simulink model "schemaSIM"  (R2015b)
settings: Solver=VariableStepAuto  StartTime=0.0  StopTime=paramSIM.T  RelTol=1e-3
undefined symbols (not defined in the file or in its folder): initENG, initEST, paramENG, paramEST, paramGPS, paramIMU, paramODO
settings Model: Creator=mouyon  LastModifiedBy=mouyon

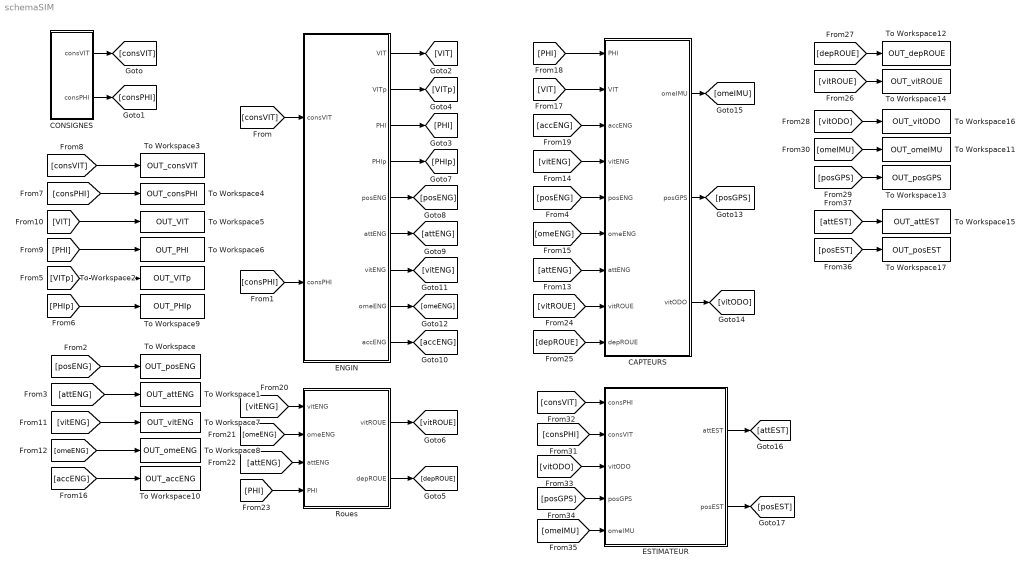
== system schemaSIM ==
  CAPTEURS : Subsystem
  CONSIGNES : Subsystem
  ENGIN : Subsystem
  ESTIMATEUR : Subsystem
  Roues : Subsystem
  To Workspace : ToWorkspace  VariableName=OUT_posENG  SaveFormat=Structure With Time  SampleTime=-1
  To Workspace1 : ToWorkspace  VariableName=OUT_attENG  SaveFormat=Structure With Time  SampleTime=-1
  To Workspace10 : ToWorkspace  VariableName=OUT_accENG  SaveFormat=Structure With Time  SampleTime=-1
  To Workspace11 : ToWorkspace  VariableName=OUT_omeIMU  SaveFormat=Structure With Time  SampleTime=-1
  To Workspace12 : ToWorkspace  VariableName=OUT_depROUE  SaveFormat=Structure With Time  SampleTime=-1
  To Workspace13 : ToWorkspace  VariableName=OUT_posGPS  SaveFormat=Structure With Time  SampleTime=-1
  To Workspace14 : ToWorkspace  VariableName=OUT_vitROUE  SaveFormat=Structure With Time  SampleTime=-1
  To Workspace15 : ToWorkspace  VariableName=OUT_attEST  SaveFormat=Structure With Time  SampleTime=-1
  To Workspace16 : ToWorkspace  VariableName=OUT_vitODO  SaveFormat=Structure With Time  SampleTime=-1
  To Workspace17 : ToWorkspace  VariableName=OUT_posEST  SaveFormat=Structure With Time  SampleTime=-1
  To Workspace2 : ToWorkspace  VariableName=OUT_VITp  SaveFormat=Structure With Time  SampleTime=-1
  To Workspace3 : ToWorkspace  VariableName=OUT_consVIT  SaveFormat=Structure With Time  SampleTime=-1
  To Workspace4 : ToWorkspace  VariableName=OUT_consPHI  SaveFormat=Structure With Time  SampleTime=-1
  To Workspace5 : ToWorkspace  VariableName=OUT_VIT  SaveFormat=Structure With Time  SampleTime=-1
  To Workspace6 : ToWorkspace  VariableName=OUT_PHI  SaveFormat=Structure With Time  SampleTime=-1
  To Workspace7 : ToWorkspace  VariableName=OUT_vitENG  SaveFormat=Structure With Time  SampleTime=-1
  To Workspace8 : ToWorkspace  VariableName=OUT_omeENG  SaveFormat=Structure With Time  SampleTime=-1
  To Workspace9 : ToWorkspace  VariableName=OUT_PHIp  SaveFormat=Structure With Time  SampleTime=-1
  wires:
  CONSIGNES/1(consVIT) -> [consVIT]
  CONSIGNES/2(consPHI) -> [consPHI]
  [consVIT] -> ENGIN/1(consVIT)
  [consPHI] -> ENGIN/2(consPHI)
  [posENG] -> To Workspace/1
  [attENG] -> To Workspace1/1
  [consVIT] -> To Workspace3/1
  [consPHI] -> To Workspace4/1
  [VIT] -> To Workspace5/1
  [PHI] -> To Workspace6/1
  [vitENG] -> To Workspace7/1
  [omeENG] -> To Workspace8/1
  ENGIN/1(VIT) -> [VIT]
  ENGIN/2(VITp) -> [VITp]
  ENGIN/3(PHI) -> [PHI]
  ENGIN/4(PHIp) -> [PHIp]
  ENGIN/6(attENG) -> [attENG]
  ENGIN/5(posENG) -> [posENG]
  ENGIN/9(accENG) -> [accENG]
  ENGIN/7(vitENG) -> [vitENG]
  [VITp] -> To Workspace2/1
  [PHIp] -> To Workspace9/1
  [accENG] -> To Workspace10/1
  [PHI] -> CAPTEURS/1(PHI)
  [VIT] -> CAPTEURS/2(VIT)
  [accENG] -> CAPTEURS/3(accENG)
  [vitENG] -> CAPTEURS/4(vitENG)
  [posENG] -> CAPTEURS/5(posENG)
  [omeENG] -> CAPTEURS/6(omeENG)
  [attENG] -> CAPTEURS/7(attENG)
  [attENG] -> Roues/3(attENG)
  [vitENG] -> Roues/1(vitENG)
  [omeENG] -> Roues/2(omeENG)
  [PHI] -> Roues/4(PHI)
  Roues/1(vitROUE) -> [vitROUE]
  Roues/2(depROUE) -> [depROUE]
  [vitROUE] -> CAPTEURS/8(vitROUE)
  [depROUE] -> CAPTEURS/9(depROUE)
  [vitROUE] -> To Workspace14/1
  [depROUE] -> To Workspace12/1
  CAPTEURS/3(vitODO) -> [vitODO]
  [vitODO] -> To Workspace16/1
  CAPTEURS/2(posGPS) -> [posGPS]
  CAPTEURS/1(omeIMU) -> [omeIMU]
  [omeIMU] -> To Workspace11/1
  ENGIN/8(omeENG) -> [omeENG]
  [posGPS] -> To Workspace13/1
  [consVIT] -> ESTIMATEUR/1(consPHI)
  [consPHI] -> ESTIMATEUR/2(consVIT)
  [vitODO] -> ESTIMATEUR/3(vitODO)
  [posGPS] -> ESTIMATEUR/4(posGPS)
  [omeIMU] -> ESTIMATEUR/5(omeIMU)
  ESTIMATEUR/1(attEST) -> [attEST]
  ESTIMATEUR/2(posEST) -> [posEST]
  [attEST] -> To Workspace15/1
  [posEST] -> To Workspace17/1

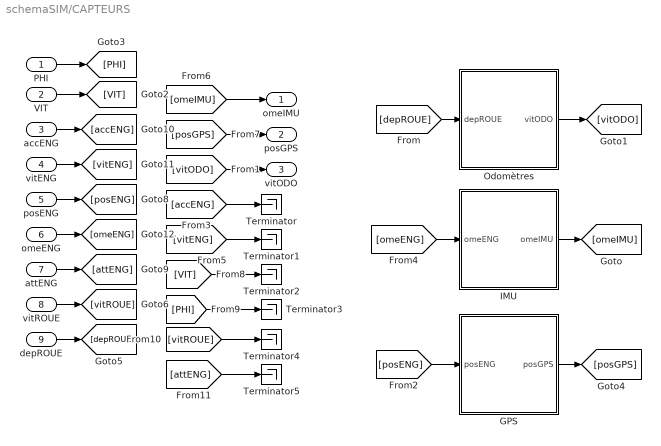
== system schemaSIM/CAPTEURS ==
  PHI : Inport
  VIT : Inport  Port=2
  accENG : Inport  Port=3
  vitENG : Inport  Port=4
  posENG : Inport  Port=5
  omeENG : Inport  Port=6
  attENG : Inport  Port=7
  vitROUE : Inport  Port=8
  depROUE : Inport  Port=9
  GPS : Subsystem
  IMU : Subsystem
  Odomètres : Subsystem
  Terminator{,1..5} (6 alike) : Terminator
  omeIMU : Outport
  posGPS : Outport  Port=2
  vitODO : Outport  Port=3
  wires:
  PHI/1 -> [PHI]
  VIT/1 -> [VIT]
  accENG/1 -> [accENG]
  vitENG/1 -> [vitENG]
  posENG/1 -> [posENG]
  omeENG/1 -> [omeENG]
  attENG/1 -> [attENG]
  vitROUE/1 -> [vitROUE]
  depROUE/1 -> [depROUE]
  [depROUE] -> Odomètres/1(depROUE)
  Odomètres/1(vitODO) -> [vitODO]
  [vitODO] -> vitODO/1
  [posGPS] -> posGPS/1
  [omeIMU] -> omeIMU/1
  [omeENG] -> IMU/1(omeENG)
  IMU/1(omeIMU) -> [omeIMU]
  [posENG] -> GPS/1(posENG)
  GPS/1(posGPS) -> [posGPS]
  [accENG] -> Terminator/1
  [vitENG] -> Terminator1/1
  [VIT] -> Terminator2/1
  [PHI] -> Terminator3/1
  [vitROUE] -> Terminator4/1
  [attENG] -> Terminator5/1

== system schemaSIM/CONSIGNES ==
  From Workspace : FromWorkspace  VariableName=IN_consVIT  SampleTime=0  Interpolate=off  OutputAfterFinalValue=Holding final value
  From Workspace1 : FromWorkspace  VariableName=IN_consPHI  SampleTime=0  Interpolate=off  OutputAfterFinalValue=Holding final value
  consVIT : Outport
  consPHI : Outport  Port=2
  wires:
  From Workspace/1 -> consVIT/1
  From Workspace1/1 -> consPHI/1

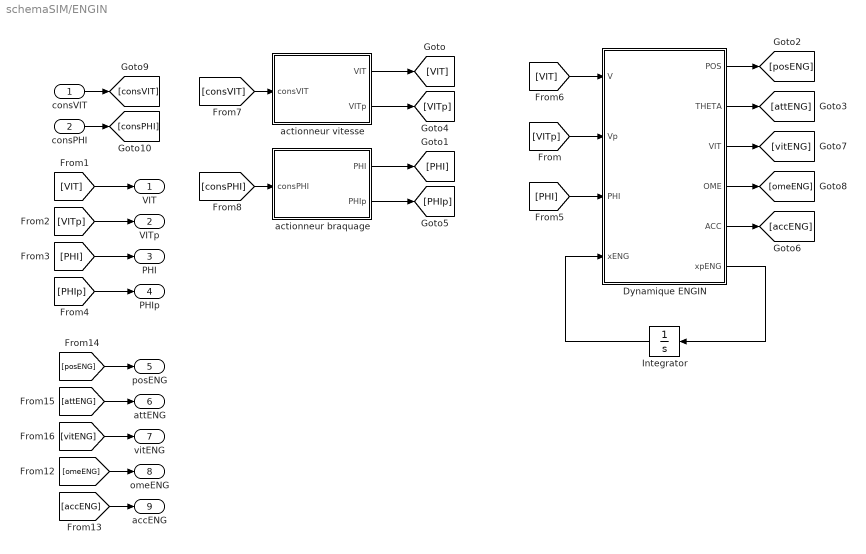
== system schemaSIM/ENGIN ==
  consVIT : Inport
  consPHI : Inport  Port=2
  Dynamique ENGIN : MATLAB Function  TreatAsAtomicUnit=on
  Integrator : Integrator  InitialCondition=initENG.x
  actionneur braquage : Subsystem
  actionneur vitesse : Subsystem
  VIT : Outport
  VITp : Outport  Port=2
  PHI : Outport  Port=3
  PHIp : Outport  Port=4
  posENG : Outport  Port=5
  attENG : Outport  Port=6
  vitENG : Outport  Port=7
  omeENG : Outport  Port=8
  accENG : Outport  Port=9
  wires:
  actionneur vitesse/1(VIT) -> [VIT]
  actionneur braquage/1(PHI) -> [PHI]
  Integrator/1 -> Dynamique ENGIN/4(xENG)
  Dynamique ENGIN/6(xpENG) -> Integrator/1
  Dynamique ENGIN/1(POS) -> [posENG]
  Dynamique ENGIN/2(THETA) -> [attENG]
  [VIT] -> Dynamique ENGIN/1(V)
  [PHI] -> Dynamique ENGIN/3(PHI)
  Dynamique ENGIN/3(VIT) -> [vitENG]
  Dynamique ENGIN/4(OME) -> [omeENG]
  actionneur vitesse/2(VITp) -> [VITp]
  actionneur braquage/2(PHIp) -> [PHIp]
  [VITp] -> Dynamique ENGIN/2(Vp)
  Dynamique ENGIN/5(ACC) -> [accENG]
  [VIT] -> VIT/1
  [VITp] -> VITp/1
  [PHI] -> PHI/1
  [PHIp] -> PHIp/1
  [posENG] -> posENG/1
  [attENG] -> attENG/1
  [vitENG] -> vitENG/1
  [omeENG] -> omeENG/1
  [accENG] -> accENG/1
  consVIT/1 -> [consVIT]
  consPHI/1 -> [consPHI]
  [consVIT] -> actionneur vitesse/1(consVIT)
  [consPHI] -> actionneur braquage/1(consPHI)

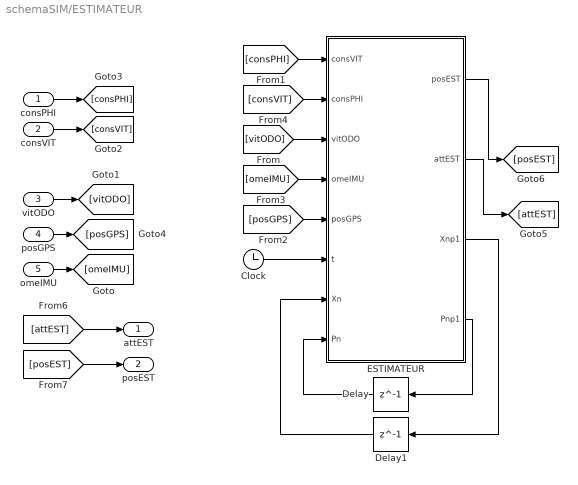
== system schemaSIM/ESTIMATEUR ==
  consPHI : Inport
  consVIT : Inport  Port=2
  vitODO : Inport  Port=3
  posGPS : Inport  Port=4
  omeIMU : Inport  Port=5
  Clock : Clock
  Delay : Delay  DelayLength=1  InitialCondition=initEST.P  SampleTime=paramEST.dt
  Delay1 : Delay  DelayLength=1  InitialCondition=initEST.x  SampleTime=paramEST.dt
  ESTIMATEUR : MATLAB Function  TreatAsAtomicUnit=on
  attEST : Outport
  posEST : Outport  Port=2
  wires:
  consPHI/1 -> [consPHI]
  consVIT/1 -> [consVIT]
  vitODO/1 -> [vitODO]
  posGPS/1 -> [posGPS]
  omeIMU/1 -> [omeIMU]
  [posEST] -> posEST/1
  [attEST] -> attEST/1
  [vitODO] -> ESTIMATEUR/3(vitODO)
  [omeIMU] -> ESTIMATEUR/4(omeIMU)
  [posGPS] -> ESTIMATEUR/5(posGPS)
  Clock/1 -> ESTIMATEUR/6(t)
  ESTIMATEUR/4(Pnp1) -> Delay/1
  ESTIMATEUR/3(Xnp1) -> Delay1/1
  ESTIMATEUR/1(posEST) -> [posEST]
  ESTIMATEUR/2(attEST) -> [attEST]
  Delay1/1 -> ESTIMATEUR/7(Xn)
  Delay/1 -> ESTIMATEUR/8(Pn)
  [consPHI] -> ESTIMATEUR/1(consVIT)
  [consVIT] -> ESTIMATEUR/2(consPHI)

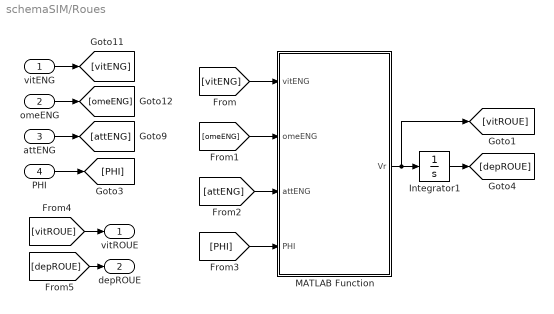
== system schemaSIM/Roues ==
  vitENG : Inport
  omeENG : Inport  Port=2
  attENG : Inport  Port=3
  PHI : Inport  Port=4
  Integrator1 : Integrator  InitialCondition=zeros(4,1)
  MATLAB Function : MATLAB Function  TreatAsAtomicUnit=on
  vitROUE : Outport
  depROUE : Outport  Port=2
  wires:
  [vitENG] -> MATLAB Function/1(vitENG)
  [omeENG] -> MATLAB Function/2(omeENG)
  [attENG] -> MATLAB Function/3(attENG)
  [PHI] -> MATLAB Function/4(PHI)
  MATLAB Function/1(Vr) -> [vitROUE], Integrator1/1
  Integrator1/1 -> [depROUE]
  vitENG/1 -> [vitENG]
  omeENG/1 -> [omeENG]
  attENG/1 -> [attENG]
  PHI/1 -> [PHI]
  [vitROUE] -> vitROUE/1
  [depROUE] -> depROUE/1

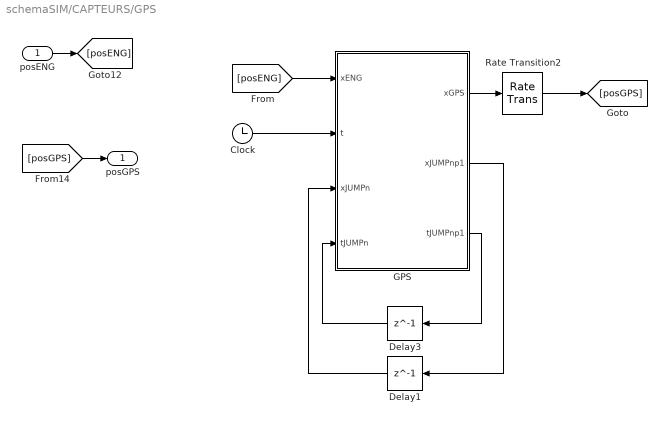
== system schemaSIM/CAPTEURS/GPS ==
  posENG : Inport
  Clock : Clock
  Delay1 : Delay  DelayLength=1  InitialCondition=zeros(2,1)  SampleTime=paramGPS.dt
  Delay3 : Delay  DelayLength=1  InitialCondition=paramGPS.per_sau*rand  SampleTime=paramGPS.dt
  GPS : MATLAB Function  TreatAsAtomicUnit=on
  Rate Transition2 : RateTransition  OutPortSampleTime=paramGPS.dt
  posGPS : Outport
  wires:
  [posGPS] -> posGPS/1
  posENG/1 -> [posENG]
  Clock/1 -> GPS/2(t)
  GPS/1(xGPS) -> Rate Transition2/1
  GPS/3(tJUMPnp1) -> Delay3/1
  Delay3/1 -> GPS/4(tJUMPn)
  GPS/2(xJUMPnp1) -> Delay1/1
  Delay1/1 -> GPS/3(xJUMPn)
  Rate Transition2/1 -> [posGPS]
  [posENG] -> GPS/1(xENG)

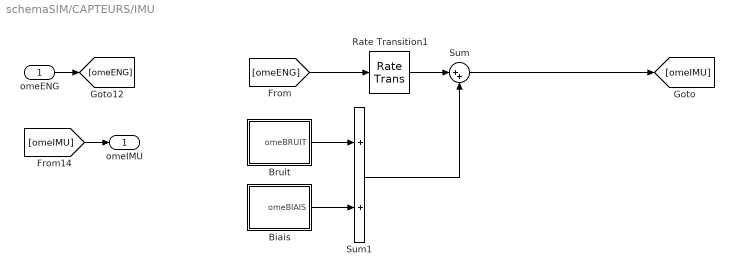
== system schemaSIM/CAPTEURS/IMU ==
  omeENG : Inport
  Biais : Subsystem
  Bruit : Subsystem
  Rate Transition1 : RateTransition  OutPortSampleTime=paramIMU.dt
  Sum : Sum  Inputs=|++
  Sum1 : Sum
  omeIMU : Outport
  wires:
  [omeIMU] -> omeIMU/1
  omeENG/1 -> [omeENG]
  [omeENG] -> Rate Transition1/1
  Rate Transition1/1 -> Sum/1
  Bruit/1(omeBRUIT) -> Sum1/1
  Biais/1(omeBIAIS) -> Sum1/2
  Sum1/1 -> Sum/2
  Sum/1 -> [omeIMU]

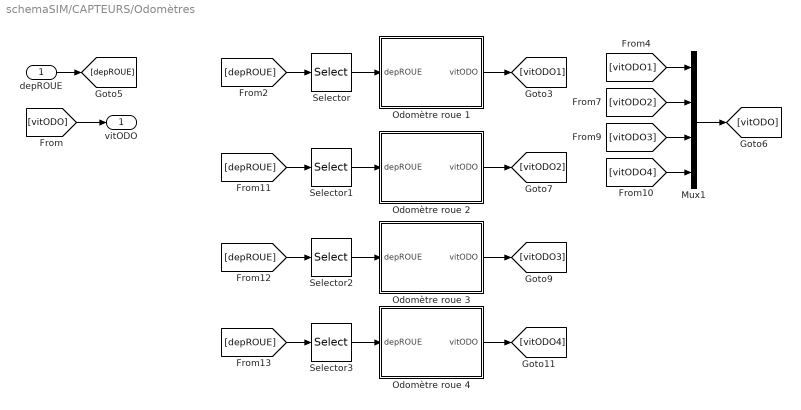
== system schemaSIM/CAPTEURS/Odomètres ==
  depROUE : Inport
  Mux1 : Mux
  Odomètre roue 1 : Subsystem
  Odomètre roue 2 : Subsystem
  Odomètre roue 3 : Subsystem
  Odomètre roue 4 : Subsystem
  Selector : Selector  InputPortWidth=4  IndexOptions=Index vector (dialog)  Indices=[1]  OutputSizes=1
  Selector1 : Selector  InputPortWidth=4  IndexOptions=Index vector (dialog)  Indices=[2]  OutputSizes=1
  Selector2 : Selector  InputPortWidth=4  IndexOptions=Index vector (dialog)  Indices=[3]  OutputSizes=1
  Selector3 : Selector  InputPortWidth=4  IndexOptions=Index vector (dialog)  Indices=[4]  OutputSizes=1
  vitODO : Outport
  wires:
  depROUE/1 -> [depROUE]
  [vitODO] -> vitODO/1
  [depROUE] -> Selector/1
  Selector/1 -> Odomètre roue 1/1(depROUE)
  Odomètre roue 1/1(vitODO) -> [vitODO1]
  Mux1/1 -> [vitODO]
  [vitODO1] -> Mux1/1
  [vitODO2] -> Mux1/2
  [vitODO3] -> Mux1/3
  [vitODO4] -> Mux1/4
  [depROUE] -> Selector1/1
  Selector1/1 -> Odomètre roue 2/1(depROUE)
  Odomètre roue 2/1(vitODO) -> [vitODO2]
  [depROUE] -> Selector2/1
  Selector2/1 -> Odomètre roue 3/1(depROUE)
  Odomètre roue 3/1(vitODO) -> [vitODO3]
  [depROUE] -> Selector3/1
  Selector3/1 -> Odomètre roue 4/1(depROUE)
  Odomètre roue 4/1(vitODO) -> [vitODO4]

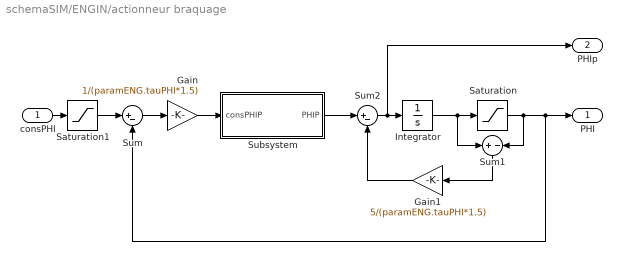
== system schemaSIM/ENGIN/actionneur braquage ==
  consPHI : Inport
  Gain : Gain  Gain=1/(paramENG.tauPHI*1.5)
  Gain1 : Gain  Gain=5/(paramENG.tauPHI*1.5)
  Integrator : Integrator  InitialCondition=initENG.PHI
  Saturation : Saturate  UpperLimit=paramENG.maxPHI  LowerLimit=-paramENG.maxPHI
  Saturation1 : Saturate  UpperLimit=paramENG.maxPHI  LowerLimit=-paramENG.maxPHI
  Subsystem : Subsystem
  Sum : Sum  Inputs=|+-
  Sum1 : Sum  Inputs=+|-
  Sum2 : Sum  Inputs=|+-
  PHI : Outport
  PHIp : Outport  Port=2
  wires:
  Integrator/1 -> Sum1/1, Saturation/1
  consPHI/1 -> Saturation1/1
  Sum/1 -> Gain/1
  Saturation/1 -> Sum1/2, PHI/1, Sum/2
  Sum1/1 -> Gain1/1
  Gain1/1 -> Sum2/2
  Sum2/1 -> PHIp/1, Integrator/1
  Gain/1 -> Subsystem/1(consPHIP)
  Subsystem/1(PHIP) -> Sum2/1
  Saturation1/1 -> Sum/1

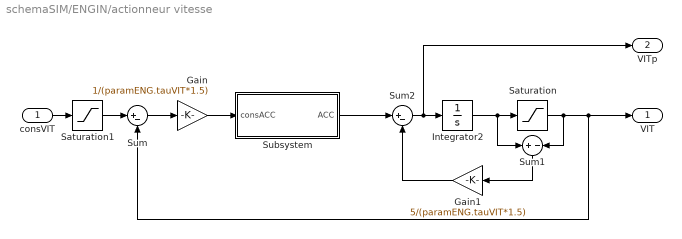
== system schemaSIM/ENGIN/actionneur vitesse ==
  consVIT : Inport
  Gain : Gain  Gain=1/(paramENG.tauVIT*1.5)
  Gain1 : Gain  Gain=5/(paramENG.tauVIT*1.5)
  Integrator2 : Integrator  InitialCondition=initENG.VIT
  Saturation : Saturate  UpperLimit=paramENG.maxVIT  LowerLimit=paramENG.minVIT
  Saturation1 : Saturate  UpperLimit=paramENG.maxVIT  LowerLimit=paramENG.minVIT
  Subsystem : Subsystem
  Sum : Sum  Inputs=|+-
  Sum1 : Sum  Inputs=+|-
  Sum2 : Sum  Inputs=|+-
  VIT : Outport
  VITp : Outport  Port=2
  wires:
  Integrator2/1 -> Sum1/1, Saturation/1
  consVIT/1 -> Saturation1/1
  Sum/1 -> Gain/1
  Saturation/1 -> Sum1/2, VIT/1, Sum/2
  Sum1/1 -> Gain1/1
  Gain1/1 -> Sum2/2
  Sum2/1 -> VITp/1, Integrator2/1
  Gain/1 -> Subsystem/1(consACC)
  Subsystem/1(ACC) -> Sum2/1
  Saturation1/1 -> Sum/1

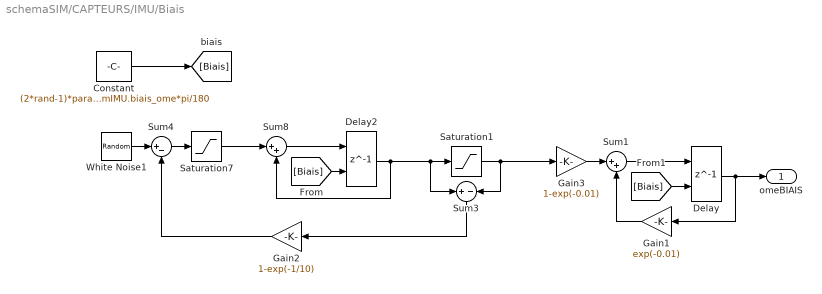
== system schemaSIM/CAPTEURS/IMU/Biais ==
  Constant : Constant  Value=(2*rand-1)*paramIMU.biais_ome*pi/180
  Delay : Delay  DelayLength=1  InitialConditionSource=Input port  InitialCondition=0
      settings: InputPortMap=u0,p4
  Delay2 : Delay  DelayLength=1  InitialConditionSource=Input port  InitialCondition=0
      settings: InputPortMap=u0,p4
  Gain1 : Gain  Gain=exp(-0.01)
  Gain2 : Gain  Gain=1-exp(-1/10)
  Gain3 : Gain  Gain=1-exp(-0.01)
  Saturation1 : Saturate  UpperLimit=paramIMU.biais_ome*pi/180  LowerLimit=-paramIMU.biais_ome*pi/180
  Saturation7 : Saturate  UpperLimit=paramIMU.deriv_ome*pi/180*paramIMU.dt  LowerLimit=-paramIMU.deriv_ome*pi/180*paramIMU.dt
  Sum1 : Sum  Inputs=|++
  Sum3 : Sum  Inputs=+|-
  Sum4 : Sum  Inputs=|+-
  Sum8 : Sum  Inputs=|++
  White Noise1 : RandomNumber  DisableCoverage=on  Variance=0.995*(paramIMU.biais_ome*pi/180/3)^2  SampleTime=paramIMU.dt
  omeBIAIS : Outport
  wires:
  Constant/1 -> [Biais]
  Delay/1 -> omeBIAIS/1, Gain1/1
  Sum1/1 -> Delay/1
  [Biais] -> Delay/2
  Gain3/1 -> Sum1/1
  Gain1/1 -> Sum1/2
  Sum3/1 -> Gain2/1
  Gain2/1 -> Sum4/2
  White Noise1/1 -> Sum4/1
  [Biais] -> Delay2/2
  Sum8/1 -> Delay2/1
  Sum4/1 -> Saturation7/1
  Delay2/1 -> Sum3/1, Saturation1/1, Sum8/2
  Saturation1/1 -> Gain3/1, Sum3/2
  Saturation7/1 -> Sum8/1

== system schemaSIM/CAPTEURS/IMU/Bruit ==
  White Noise : RandomNumber  DisableCoverage=on  Variance=(paramIMU.sig_ome*pi/180)^2  SampleTime=paramIMU.dt
  omeBRUIT : Outport
  wires:
  White Noise/1 -> omeBRUIT/1

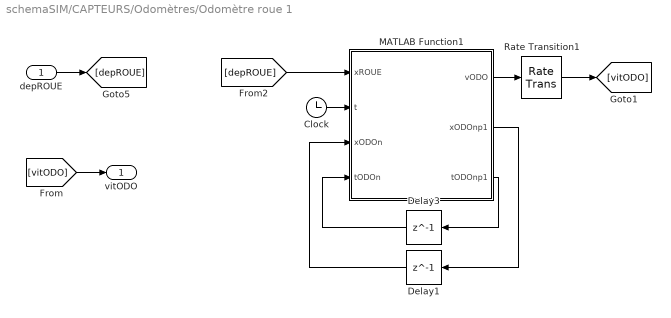
== system schemaSIM/CAPTEURS/Odomètres/Odomètre roue 1 ==
  depROUE : Inport
  Clock : Clock
  Delay1 : Delay  DelayLength=1  InitialCondition=0  SampleTime=paramODO.dt
  Delay3 : Delay  DelayLength=1  InitialCondition=0  SampleTime=paramODO.dt
  MATLAB Function1 : MATLAB Function  TreatAsAtomicUnit=on
  Rate Transition1 : RateTransition  OutPortSampleTime=paramODO.dt
  vitODO : Outport
  wires:
  Clock/1 -> MATLAB Function1/2(t)
  MATLAB Function1/1(vODO) -> Rate Transition1/1
  Rate Transition1/1 -> [vitODO]
  MATLAB Function1/3(tODOnp1) -> Delay3/1
  Delay3/1 -> MATLAB Function1/4(tODOn)
  MATLAB Function1/2(xODOnp1) -> Delay1/1
  Delay1/1 -> MATLAB Function1/3(xODOn)
  depROUE/1 -> [depROUE]
  [depROUE] -> MATLAB Function1/1(xROUE)
  [vitODO] -> vitODO/1

== system schemaSIM/CAPTEURS/Odomètres/Odomètre roue 2 ==
  depROUE : Inport
  Clock : Clock
  Delay1 : Delay  DelayLength=1  InitialCondition=0  SampleTime=paramODO.dt
  Delay3 : Delay  DelayLength=1  InitialCondition=0  SampleTime=paramODO.dt
  MATLAB Function1 : MATLAB Function  TreatAsAtomicUnit=on
  Rate Transition1 : RateTransition  OutPortSampleTime=paramODO.dt
  vitODO : Outport
  wires:
  Clock/1 -> MATLAB Function1/2(t)
  MATLAB Function1/1(vODO) -> Rate Transition1/1
  Rate Transition1/1 -> [vitODO]
  MATLAB Function1/3(tODOnp1) -> Delay3/1
  Delay3/1 -> MATLAB Function1/4(tODOn)
  MATLAB Function1/2(xODOnp1) -> Delay1/1
  Delay1/1 -> MATLAB Function1/3(xODOn)
  depROUE/1 -> [depROUE]
  [depROUE] -> MATLAB Function1/1(xROUE)
  [vitODO] -> vitODO/1

== system schemaSIM/CAPTEURS/Odomètres/Odomètre roue 3 ==
  depROUE : Inport
  Clock : Clock
  Delay1 : Delay  DelayLength=1  InitialCondition=0  SampleTime=paramODO.dt
  Delay3 : Delay  DelayLength=1  InitialCondition=0  SampleTime=paramODO.dt
  MATLAB Function1 : MATLAB Function  TreatAsAtomicUnit=on
  Rate Transition1 : RateTransition  OutPortSampleTime=paramODO.dt
  vitODO : Outport
  wires:
  Clock/1 -> MATLAB Function1/2(t)
  MATLAB Function1/1(vODO) -> Rate Transition1/1
  Rate Transition1/1 -> [vitODO]
  MATLAB Function1/3(tODOnp1) -> Delay3/1
  Delay3/1 -> MATLAB Function1/4(tODOn)
  MATLAB Function1/2(xODOnp1) -> Delay1/1
  Delay1/1 -> MATLAB Function1/3(xODOn)
  depROUE/1 -> [depROUE]
  [depROUE] -> MATLAB Function1/1(xROUE)
  [vitODO] -> vitODO/1

== system schemaSIM/CAPTEURS/Odomètres/Odomètre roue 4 ==
  depROUE : Inport
  Clock : Clock
  Delay1 : Delay  DelayLength=1  InitialCondition=0  SampleTime=paramODO.dt
  Delay3 : Delay  DelayLength=1  InitialCondition=0  SampleTime=paramODO.dt
  MATLAB Function1 : MATLAB Function  TreatAsAtomicUnit=on
  Rate Transition1 : RateTransition  OutPortSampleTime=paramODO.dt
  vitODO : Outport
  wires:
  Clock/1 -> MATLAB Function1/2(t)
  MATLAB Function1/1(vODO) -> Rate Transition1/1
  Rate Transition1/1 -> [vitODO]
  MATLAB Function1/3(tODOnp1) -> Delay3/1
  Delay3/1 -> MATLAB Function1/4(tODOn)
  MATLAB Function1/2(xODOnp1) -> Delay1/1
  Delay1/1 -> MATLAB Function1/3(xODOn)
  depROUE/1 -> [depROUE]
  [depROUE] -> MATLAB Function1/1(xROUE)
  [vitODO] -> vitODO/1

== system schemaSIM/ENGIN/actionneur braquage/Subsystem ==
  consPHIP : Inport
  Gain2 : Gain  Gain=5/(paramENG.tauPHI/1.5)
  Gain3 : Gain  Gain=1/(paramENG.tauPHI/1.5)
  Integrator1 : Integrator
  Saturation1 : Saturate  UpperLimit=paramENG.maxPHIP  LowerLimit=-paramENG.maxPHIP
  Saturation2 : Saturate  UpperLimit=paramENG.maxPHIP  LowerLimit=-paramENG.maxPHIP
  Sum3 : Sum  Inputs=+|-
  Sum4 : Sum  Inputs=|+-
  Sum5 : Sum  Inputs=|+-
  PHIP : Outport
  wires:
  Integrator1/1 -> Sum3/1, Saturation1/1
  Sum3/1 -> Gain2/1
  Gain2/1 -> Sum4/2
  Sum4/1 -> Integrator1/1
  Gain3/1 -> Sum4/1
  Saturation1/1 -> PHIP/1, Sum5/2, Sum3/2
  Sum5/1 -> Gain3/1
  consPHIP/1 -> Saturation2/1
  Saturation2/1 -> Sum5/1

== system schemaSIM/ENGIN/actionneur vitesse/Subsystem ==
  consACC : Inport
  Gain2 : Gain  Gain=5/(paramENG.tauVIT/1.5)
  Gain3 : Gain  Gain=1/(paramENG.tauVIT/1.5)
  Integrator1 : Integrator
  Saturation1 : Saturate  UpperLimit=paramENG.maxVITP  LowerLimit=-paramENG.maxVITP
  Saturation2 : Saturate  UpperLimit=paramENG.maxVITP  LowerLimit=-paramENG.maxVITP
  Sum3 : Sum  Inputs=+|-
  Sum4 : Sum  Inputs=|+-
  Sum5 : Sum  Inputs=|+-
  ACC : Outport
  wires:
  Integrator1/1 -> Sum3/1, Saturation1/1
  Sum3/1 -> Gain2/1
  Gain2/1 -> Sum4/2
  Sum4/1 -> Integrator1/1
  Gain3/1 -> Sum4/1
  Saturation1/1 -> ACC/1, Sum5/2, Sum3/2
  Sum5/1 -> Gain3/1
  consACC/1 -> Saturation2/1
  Saturation2/1 -> Sum5/1

== matlab function schemaSIM/CAPTEURS/Odomètres/Odomètre roue 2/MATLAB Function1 ==
  data: xROUE input size=1; t input size=1; xODOn input size=1; tODOn input size=1; vODO output size=1; xODOnp1 output size=1; paramODO parameter; tODOnp1 output size=1
function [vODO,xODOnp1,tODOnp1]  = Odometre(xROUE,t,xODOn,tODOn,paramODO)

% [vODO,xODOnp1,tODOnp1]  = Odometre(xROUE,t,xODOn,tODOn,paramODO);
%--------------------------------------------------------------------------
%   xROUE :	position courante de la roue 
%   t :     date courante
%   xODOn :	position au top précédent
%   tODOn :	date au top précédent
% 
%   vitODO :    vitesse mesurée 
%   xODOnp1 :	position au dernier top 
%   tODOnp1 :	date au dernier top
%--------------------------------------------------------------------------

% Paramètres
dx	= paramODO.dx;
sig	= paramODO.sig_vit;

% Variations
Dx = xROUE-xODOn;
Dt = t-tODOn;

% Incrément du nombre de TOP
nTOP = fix(Dx/dx);

% Déplacement quantifié (pas dx)
dxODO = nTOP*dx;

% Ajout incertitude de mesure
dxINC = sig*Dt*randn;
dxODO = dxODO + dxINC;

% Déplacement mesuré
if nTOP~=0
    % Au moins un TOP reçu
    xODOnp1 = xODOn + dxODO;
    tODOnp1  = t;
else
    % Aucun TOP reçu
    xODOnp1 = xODOn;
    tODOnp1 = tODOn;
end;

% Vitesse mesurée
vODO = (xODOnp1-xODOn)*Dt/(Dt*Dt+eps);

== matlab function schemaSIM/CAPTEURS/Odomètres/Odomètre roue 1/MATLAB Function1 ==
  data: xROUE input size=1; t input size=1; xODOn input size=1; tODOn input size=1; vODO output size=1; xODOnp1 output size=1; paramODO parameter; tODOnp1 output size=1
function [vODO,xODOnp1,tODOnp1]  = Odometre(xROUE,t,xODOn,tODOn,paramODO)

% [vODO,xODOnp1,tODOnp1]  = Odometre(xROUE,t,xODOn,tODOn,paramODO);
%--------------------------------------------------------------------------
%   xROUE :	position courante de la roue 
%   t :     date courante
%   xODOn :	position au top précédent
%   tODOn :	date au top précédent
% 
%   vitODO :    vitesse mesurée 
%   xODOnp1 :	position au dernier top 
%   tODOnp1 :	date au dernier top
%--------------------------------------------------------------------------

% Paramètres
dx	= paramODO.dx;
sig	= paramODO.sig_vit;

% Variations
Dx = xROUE-xODOn;
Dt = t-tODOn;

% Incrément du nombre de TOP
nTOP = fix(Dx/dx);

% Déplacement quantifié (pas dx)
dxODO = nTOP*dx;

% Ajout incertitude de mesure
dxINC = sig*Dt*randn;
dxODO = dxODO + dxINC;

% Déplacement mesuré
if nTOP~=0
    % Au moins un TOP reçu
    xODOnp1 = xODOn + dxODO;
    tODOnp1  = t;
else
    % Aucun TOP reçu
    xODOnp1 = xODOn;
    tODOnp1 = tODOn;
end;

% Vitesse mesurée
vODO = (xODOnp1-xODOn)*Dt/(Dt*Dt+eps);

== matlab function schemaSIM/ENGIN/Dynamique ENGIN ==
  data: V input size=1; Vp input; POS output size=2; THETA output size=1; VIT output; OME output; ACC output; PHI input size=1; xENG input size=initENG.nx; xpENG output size=initENG.nx; paramENG parameter
function [POS,THETA,VIT,OME,ACC,xpENG] = dynENGIN(V,Vp,PHI,xENG,paramENG)

% [POS,THETA,VIT,OME,ACC,xpENG] = dynENGIN(V,Vp,PHI,xENG,paramENG);
%--------------------------------------------------------------------------
% POS: position centre essieu arrière
% THETA: cap
% VIT: vitesse du centre de l'essieu arrière
% OME: vitesse de rotation
% ACC: accélération du centre de l'essieu arrière
%--------------------------------------------------------------------------
% WARNING: PHI est en degrés 
%--------------------------------------------------------------------------

% Decodage des arguments d'entree
x       = xENG(1);  % [m]
y       = xENG(2);  % [m]
the     = xENG(3);  % [rd]
phi     = PHI*pi/180;

% Dynamique de l'état
xp      = V * cos(the);
yp      = V * sin(the);
attp	= V/paramENG.L * tan(phi);

% Accélération
Vxp     = Vp * cos(the) - V^2 * tan(phi) * sin(the);
Vyp     = Vp * sin(the) + V^2 * tan(phi) * cos(the);

% Encodage des arguments de sortie
POS     = [x;y];
THETA	= [the];
VIT     = [xp;yp];
OME     = [attp];
ACC     = [Vxp;Vyp];
xpENG	= [xp;yp;attp];

== matlab function schemaSIM/CAPTEURS/Odomètres/Odomètre roue 3/MATLAB Function1 ==
  data: xROUE input size=1; t input size=1; xODOn input size=1; tODOn input size=1; vODO output size=1; xODOnp1 output size=1; paramODO parameter; tODOnp1 output size=1
function [vODO,xODOnp1,tODOnp1]  = Odometre(xROUE,t,xODOn,tODOn,paramODO)

% [vODO,xODOnp1,tODOnp1]  = Odometre(xROUE,t,xODOn,tODOn,paramODO);
%--------------------------------------------------------------------------
%   xROUE :	position courante de la roue 
%   t :     date courante
%   xODOn :	position au top précédent
%   tODOn :	date au top précédent
% 
%   vitODO :    vitesse mesurée 
%   xODOnp1 :	position au dernier top 
%   tODOnp1 :	date au dernier top
%--------------------------------------------------------------------------

% Paramètres
dx	= paramODO.dx;
sig	= paramODO.sig_vit;

% Variations
Dx = xROUE-xODOn;
Dt = t-tODOn;

% Incrément du nombre de TOP
nTOP = fix(Dx/dx);

% Déplacement quantifié (pas dx)
dxODO = nTOP*dx;

% Ajout incertitude de mesure
dxINC = sig*Dt*randn;
dxODO = dxODO + dxINC;

% Déplacement mesuré
if nTOP~=0
    % Au moins un TOP reçu
    xODOnp1 = xODOn + dxODO;
    tODOnp1  = t;
else
    % Aucun TOP reçu
    xODOnp1 = xODOn;
    tODOnp1 = tODOn;
end;

% Vitesse mesurée
vODO = (xODOnp1-xODOn)*Dt/(Dt*Dt+eps);

== matlab function schemaSIM/CAPTEURS/Odomètres/Odomètre roue 4/MATLAB Function1 ==
  data: xROUE input size=1; t input size=1; xODOn input size=1; tODOn input size=1; vODO output size=1; xODOnp1 output size=1; paramODO parameter; tODOnp1 output size=1
function [vODO,xODOnp1,tODOnp1]  = Odometre(xROUE,t,xODOn,tODOn,paramODO)

% [vODO,xODOnp1,tODOnp1]  = Odometre(xROUE,t,xODOn,tODOn,paramODO);
%--------------------------------------------------------------------------
%   xROUE :	position courante de la roue 
%   t :     date courante
%   xODOn :	position au top précédent
%   tODOn :	date au top précédent
% 
%   vitODO :    vitesse mesurée 
%   xODOnp1 :	position au dernier top 
%   tODOnp1 :	date au dernier top
%--------------------------------------------------------------------------

% Paramètres
dx	= paramODO.dx;
sig	= paramODO.sig_vit;

% Variations
Dx = xROUE-xODOn;
Dt = t-tODOn;

% Incrément du nombre de TOP
nTOP = fix(Dx/dx);

% Déplacement quantifié (pas dx)
dxODO = nTOP*dx;

% Ajout incertitude de mesure
dxINC = sig*Dt*randn;
dxODO = dxODO + dxINC;

% Déplacement mesuré
if nTOP~=0
    % Au moins un TOP reçu
    xODOnp1 = xODOn + dxODO;
    tODOnp1  = t;
else
    % Aucun TOP reçu
    xODOnp1 = xODOn;
    tODOnp1 = tODOn;
end;

% Vitesse mesurée
vODO = (xODOnp1-xODOn)*Dt/(Dt*Dt+eps);

== matlab function schemaSIM/Roues/MATLAB Function ==
  data: vitENG input size=2; omeENG input size=1; Vr output size=4; attENG input size=1; PHI input size=1; paramENG parameter
function Vr  = vitROUE(vitENG,omeENG,attENG,PHI,paramENG)

% Vr = vitROUE(vitENG,omeENG,attENG,PHI,paramENG);
%--------------------------------------------------------------------------
% Vr(1): vitesse roue arrière gauche
% Vr(2): vitesse roue arrière droite
% Vr(3): vitesse roue avant gauche
% Vr(4): vitesse roue avant droite
%--------------------------------------------------------------------------
% WARNING: PHI est en degrés 
%--------------------------------------------------------------------------

% Decodage des arguments d'entree
Vx      = vitENG(1);
Vy      = vitENG(2);
omega	= omeENG;
theta	= attENG;
phi     = PHI*pi/180;

% Paramètres
H   = paramENG.H;
L	= paramENG.L;

% Vitesses (de roulement) des roues
Vr = zeros(4,1);
Vr(1,1) = cos(theta)*Vx + sin(theta)*Vy - omega*H;
Vr(2,1) = cos(theta)*Vx + sin(theta)*Vy + omega*H;
Vr(3,1) = cos(theta+phi)*Vx + sin(theta+phi)*Vy - omega*(H*cos(phi)-L*sin(phi));
Vr(4,1) = cos(theta+phi)*Vx + sin(theta+phi)*Vy + omega*(H*cos(phi)+L*sin(phi));

== matlab function schemaSIM/ESTIMATEUR/ESTIMATEUR ==
  data: consVIT input; consPHI input; vitODO input size=4; omeIMU input size=1; posGPS input size=2; posEST output size=2; t input size=1; Xn input size=initEST.nx; attEST output size=1; Xnp1 output size=initEST.nx; Pn input size=[initEST.nx,initEST.nx]; paramEST parameter; Pnp1 output size=[initEST.nx,initEST.nx]
function [posEST,attEST,Xnp1,Pnp1]  = FILTRE(consVIT,consPHI,vitODO,omeIMU,posGPS,t,Xn,Pn,paramEST)

% [posEST,attEST,Xnp1,Pnp1]  = FILTRE(vitODO,omeIMU,posGPS,t,Xn,Pn,paramEST);
%--------------------------------------------------------------------------
%   consVIT :   consigne de vitesse
%   consPHI :   consigne de cap
%   vitODO :	mesure des vitesses des roues par ODOMETRE [100 Hz]
%   omeIMU :	mesure de la vitesse de rotation par IMU [100 Hz]
%   posGPS :	mesure de la position par GPS [1 Hz]
%   t :         date courante
%   Xn :        état estimé
%   Pn :        covariance de l'erreur d'estimation d'état
% 
%   posEST :    position estimée 
%   attEST :	attitude estimée 
%   Xnp1 :  	état estimé
%   Pnp1 :  	covariance de l'erreur d'estimation d'état
%--------------------------------------------------------------------------

% Paramètres
dt  = paramEST.dt;
Q   = paramEST.Q;
R   = paramEST.R;

% Décodage des entrées
x   = Xn(1,1);
y	= Xn(2,1);
the = Xn(3,1);

% Initialisation
Xnp1   = Xn;
Pnp1   = Pn;

%--------------------------------------------------------------------------
% Prédiction
%--------------------------------------------------------------------------

%--------------------------------------------------------------------------
% Correction
%--------------------------------------------------------------------------

%--------------------------------------------------------------------------
% Codage des sorties
%--------------------------------------------------------------------------
posEST = [x;y];
attEST = the;

== matlab function schemaSIM/CAPTEURS/GPS/GPS ==
  data: xENG input size=2; xGPS output size=2; t input size=1; xJUMPn input size=2; tJUMPn input size=1; paramGPS parameter; xJUMPnp1 output size=2; tJUMPnp1 output size=1
function [xGPS,xJUMPnp1,tJUMPnp1]  = GPS(xENG,t,xJUMPn,tJUMPn,paramGPS)

% [vODO,xODOnp1,tODOnp1]  = Odometre(xROUE,t,xODOn,tODOn,paramODO);
%--------------------------------------------------------------------------
%   xENG :	position courante de l'engin
%   t :     date courante
%   xJUMPn :	intégrale des sauts précédents
%   tJUMPn :	date du prochain saut
% 
%   xGPS :    position mesurée 
%   xJUMPnp1 :	intégrale des sauts  
%   tJUMPnp1 :	date au dernier saut
%--------------------------------------------------------------------------

% Paramètres
sig	= paramGPS.sig_pos;
per	= paramGPS.per_sau;
amp = paramGPS.amp_sau;

% Variations
Dt = t-tJUMPn;

% Saut à des instants Poissoniens
if Dt>=0
    % amplitude aléatoire, et retour vers zéro
%     dxGPS = -rand*xJUMPn + amp * randn(2,1);
    dxGPS = amp * (2*rand(2,1)-ones(2,1));
    dxGPS = dxGPS - exp(-0.1)*xJUMPn;
    xJUMPnp1 = xJUMPn + dxGPS; 
    % Saturation du cumul 
    xJUMPnp1(1,1) = max(-amp,min(amp,xJUMPnp1(1,1)));    
    xJUMPnp1(2,1) = max(-amp,min(amp,xJUMPnp1(2,1)));   
    % Date du prochain saut
    dt = -per*log(1-rand);
    tJUMPnp1 = t + dt;
else
    tJUMPnp1 = tJUMPn;
    xJUMPnp1 = xJUMPn;
end;

% Position mesurée 
xGPS = xENG + xJUMPnp1 + sig*randn(2,1);
